simulink model "LOG_DATI_GPS_BMP_prova"  (R2020b)
settings: Solver=ode4  StartTime=0.0  StopTime=Inf  FixedStep=0.02  RelTol=1e-3  EnableMultiTasking=on
PostLoadFcn:
  | , if any(exist('dsrtsu_mdlpostloadfcn', 'file') == [2, 3, 6]), try dsrtsu_mdlpostloadfcn('Execute', bdroot); catch fprintf('Error in PostLoadFcn (dsrtsu_mdlpostloadfcn) for model "%s":\n %s\n', bdroot, lasterr); end, end,
InitFcn:
  | , if any(exist('rtifpga_mdlclblib', 'file') ~= 0), rtifpga_mdlclblib('Init', bdroot); end,
values from neighbouring files (symbols this model uses):
  t_AP = 0.02    [AVVIO_AENEA_DATA.m]    (also in workspace_SFT.mat)
libraries: arduinolib x21, simulink_extras x6, svdutilitieslib x4, simulink x2
(part 2 of 3)

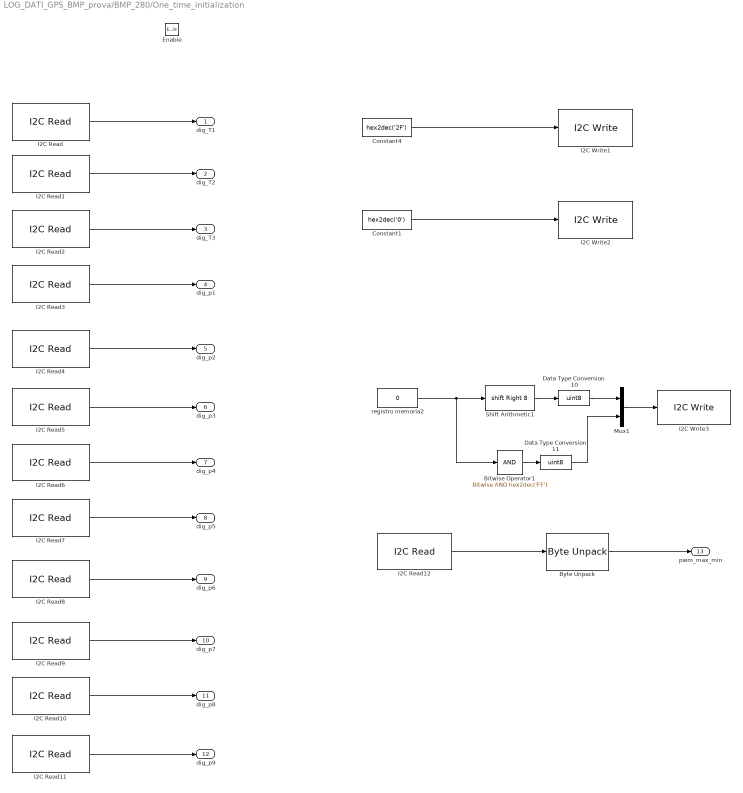
== system LOG_DATI_GPS_BMP_prova/BMP_280/One_time_initialization ==
  Enable : EnablePort
  Bitwise Operator1 : simulink/Logic and Bit Operations/Bitwise Operator  logicop=AND  UseBitMask=on  BitMask=hex2dec('FF')  BitMaskRealWorld=Stored Integer
  Byte Unpack : svdutilitieslib/Byte Unpack  dimensions={[8]}  datatypes={'uint16'}  byteAlign=1  blockPlatform=arduinoert
      settings: SourceProductBaseCode=ARDUINO
  Constant1 : Constant  Value=hex2dec('0')  OutDataTypeStr=uint8  SampleTime=-1
  Constant4 : Constant  Value=hex2dec('2F')  OutDataTypeStr=uint8  SampleTime=-1
  Data Type Conversion10 : DataTypeConversion  OutDataTypeStr=uint8
  Data Type Conversion11 : DataTypeConversion  OutDataTypeStr=uint8
  I2C Read : arduinolib/I2C Read  Priority=1  I2CModule=0  Mode=Master  SlaveAddress=hex2dec( '76' )  SlaveByteOrder=LittleEndian  Direction=Receiver  RegisterAddressMode=on  RegisterAddress=hex2dec( '88' )  SlaveDataType=uint16  DataLength=1  NoAck=off  RepeatedStart=off  OutputStatus=off  blockPlatform=arduino  SampleTime=t_AP
      settings: AttributesFormatString=Priority=%<Priority>  SourceProductBaseCode=ARDUINO
  I2C Read1 : arduinolib/I2C Read  Priority=2  I2CModule=0  Mode=Master  SlaveAddress=hex2dec( '76' )  SlaveByteOrder=LittleEndian  Direction=Receiver  RegisterAddressMode=on  RegisterAddress=hex2dec( '8A' )  SlaveDataType=int16  DataLength=1  NoAck=off  RepeatedStart=off  OutputStatus=off  blockPlatform=arduino  SampleTime=t_AP
      settings: AttributesFormatString=Priority=%<Priority>  SourceProductBaseCode=ARDUINO
  I2C Read10 : arduinolib/I2C Read  Priority=11  I2CModule=0  Mode=Master  SlaveAddress=hex2dec( '76' )  SlaveByteOrder=LittleEndian  Direction=Receiver  RegisterAddressMode=on  RegisterAddress=hex2dec( '9C' )  SlaveDataType=int16  DataLength=1  NoAck=off  RepeatedStart=off  OutputStatus=off  blockPlatform=arduino  SampleTime=t_AP
      settings: AttributesFormatString=Priority=%<Priority>  SourceProductBaseCode=ARDUINO
  I2C Read11 : arduinolib/I2C Read  Priority=12  I2CModule=0  Mode=Master  SlaveAddress=hex2dec( '76' )  SlaveByteOrder=LittleEndian  Direction=Receiver  RegisterAddressMode=on  RegisterAddress=hex2dec( '9E' )  SlaveDataType=int16  DataLength=1  NoAck=off  RepeatedStart=off  OutputStatus=off  blockPlatform=arduino  SampleTime=t_AP
      settings: AttributesFormatString=Priority=%<Priority>  SourceProductBaseCode=ARDUINO
  I2C Read12 : arduinolib/I2C Read  Priority=16  I2CModule=0  Mode=Master  SlaveAddress=hex2dec( '50' )  SlaveByteOrder=BigEndian  Direction=Receiver  RegisterAddressMode=off  RegisterAddress=0  SlaveDataType=uint8  DataLength=16  NoAck=off  RepeatedStart=off  OutputStatus=off  blockPlatform=ARDUINO  SampleTime=0.02
      settings: AttributesFormatString=Priority=%<Priority>  SourceProductBaseCode=ARDUINO
  I2C Read2 : arduinolib/I2C Read  Priority=3  I2CModule=0  Mode=Master  SlaveAddress=hex2dec( '76' )  SlaveByteOrder=LittleEndian  Direction=Receiver  RegisterAddressMode=on  RegisterAddress=hex2dec( '8C' )  SlaveDataType=int16  DataLength=1  NoAck=off  RepeatedStart=off  OutputStatus=off  blockPlatform=arduino  SampleTime=t_AP
      settings: AttributesFormatString=Priority=%<Priority>  SourceProductBaseCode=ARDUINO
  I2C Read3 : arduinolib/I2C Read  Priority=4  I2CModule=0  Mode=Master  SlaveAddress=hex2dec( '76' )  SlaveByteOrder=LittleEndian  Direction=Receiver  RegisterAddressMode=on  RegisterAddress=hex2dec( '8E' )  SlaveDataType=uint16  DataLength=1  NoAck=off  RepeatedStart=off  OutputStatus=off  blockPlatform=arduino  SampleTime=t_AP
      settings: AttributesFormatString=Priority=%<Priority>  SourceProductBaseCode=ARDUINO
  I2C Read4 : arduinolib/I2C Read  Priority=5  I2CModule=0  Mode=Master  SlaveAddress=hex2dec( '76' )  SlaveByteOrder=LittleEndian  Direction=Receiver  RegisterAddressMode=on  RegisterAddress=hex2dec( '90' )  SlaveDataType=int16  DataLength=1  NoAck=off  RepeatedStart=off  OutputStatus=off  blockPlatform=arduino  SampleTime=t_AP
      settings: AttributesFormatString=Priority=%<Priority>  SourceProductBaseCode=ARDUINO
  I2C Read5 : arduinolib/I2C Read  Priority=6  I2CModule=0  Mode=Master  SlaveAddress=hex2dec( '76' )  SlaveByteOrder=LittleEndian  Direction=Receiver  RegisterAddressMode=on  RegisterAddress=hex2dec( '92' )  SlaveDataType=int16  DataLength=1  NoAck=off  RepeatedStart=off  OutputStatus=off  blockPlatform=arduino  SampleTime=t_AP
      settings: AttributesFormatString=Priority=%<Priority>  SourceProductBaseCode=ARDUINO
  I2C Read6 : arduinolib/I2C Read  Priority=7  I2CModule=0  Mode=Master  SlaveAddress=hex2dec( '76' )  SlaveByteOrder=LittleEndian  Direction=Receiver  RegisterAddressMode=on  RegisterAddress=hex2dec( '94' )  SlaveDataType=int16  DataLength=1  NoAck=off  RepeatedStart=off  OutputStatus=off  blockPlatform=arduino  SampleTime=t_AP
      settings: AttributesFormatString=Priority=%<Priority>  SourceProductBaseCode=ARDUINO
  I2C Read7 : arduinolib/I2C Read  Priority=8  I2CModule=0  Mode=Master  SlaveAddress=hex2dec( '76' )  SlaveByteOrder=LittleEndian  Direction=Receiver  RegisterAddressMode=on  RegisterAddress=hex2dec( '96' )  SlaveDataType=int16  DataLength=1  NoAck=off  RepeatedStart=off  OutputStatus=off  blockPlatform=arduino  SampleTime=t_AP
      settings: AttributesFormatString=Priority=%<Priority>  SourceProductBaseCode=ARDUINO
  I2C Read8 : arduinolib/I2C Read  Priority=9  I2CModule=0  Mode=Master  SlaveAddress=hex2dec( '76' )  SlaveByteOrder=LittleEndian  Direction=Receiver  RegisterAddressMode=on  RegisterAddress=hex2dec( '98' )  SlaveDataType=int16  DataLength=1  NoAck=off  RepeatedStart=off  OutputStatus=off  blockPlatform=arduino  SampleTime=t_AP
      settings: AttributesFormatString=Priority=%<Priority>  SourceProductBaseCode=ARDUINO
  I2C Read9 : arduinolib/I2C Read  Priority=10  I2CModule=0  Mode=Master  SlaveAddress=hex2dec( '76' )  SlaveByteOrder=LittleEndian  Direction=Receiver  RegisterAddressMode=on  RegisterAddress=hex2dec( '9A' )  SlaveDataType=int16  DataLength=1  NoAck=off  RepeatedStart=off  OutputStatus=off  blockPlatform=arduino  SampleTime=t_AP
      settings: AttributesFormatString=Priority=%<Priority>  SourceProductBaseCode=ARDUINO
  I2C Write1 : arduinolib/I2C Write  Priority=13  I2CModule=0  Mode=Master  SlaveAddress=hex2dec( '76' )  SlaveByteOrder=LittleEndian  Direction=Transmitter  RegisterAddressMode=on  RegisterAddress=hex2dec( 'F4' )  SlaveDataType=uint8  DataLength=1  NoAck=off  RepeatedStart=off  OutputStatus=off  blockPlatform=arduino
      settings: AttributesFormatString=Priority=%<Priority>  SourceProductBaseCode=ARDUINO
  I2C Write2 : arduinolib/I2C Write  Priority=14  I2CModule=0  Mode=Master  SlaveAddress=hex2dec( '76' )  SlaveByteOrder=LittleEndian  Direction=Transmitter  RegisterAddressMode=on  RegisterAddress=hex2dec( 'F5' )  SlaveDataType=uint8  DataLength=1  NoAck=off  RepeatedStart=off  OutputStatus=off  blockPlatform=arduino
      settings: AttributesFormatString=Priority=%<Priority>  SourceProductBaseCode=ARDUINO
  I2C Write3 : arduinolib/I2C Write  Priority=15  I2CModule=0  Mode=Master  SlaveAddress=hex2dec( '50' )  SlaveByteOrder=BigEndian  Direction=Transmitter  RegisterAddressMode=off  RegisterAddress=hex2dec( '0' )  SlaveDataType=uint8  DataLength=1  NoAck=off  RepeatedStart=off  OutputStatus=off  blockPlatform=ARDUINO
      settings: AttributesFormatString=Priority=%<Priority>  SourceProductBaseCode=ARDUINO
  Mux1 : Mux  Inputs=2
  Shift Arithmetic1 : ArithShift  BitShiftNumber=8  BitShiftDirection=Right
  "registro memoria2 " : Constant  Value=0  OutDataTypeStr=uint16  SampleTime=t_AP
  dig_T1 : Outport  VectorParamsAs1DForOutWhenUnconnected=off
  dig_T2 : Outport  Port=2  VectorParamsAs1DForOutWhenUnconnected=off
  dig_T3 : Outport  Port=3  VectorParamsAs1DForOutWhenUnconnected=off
  dig_p1 : Outport  Port=4  VectorParamsAs1DForOutWhenUnconnected=off
  dig_p2 : Outport  Port=5  VectorParamsAs1DForOutWhenUnconnected=off
  dig_p3 : Outport  Port=6  VectorParamsAs1DForOutWhenUnconnected=off
  dig_p4 : Outport  Port=7  VectorParamsAs1DForOutWhenUnconnected=off
  dig_p5 : Outport  Port=8  VectorParamsAs1DForOutWhenUnconnected=off
  dig_p6 : Outport  Port=9  VectorParamsAs1DForOutWhenUnconnected=off
  dig_p7 : Outport  Port=10  VectorParamsAs1DForOutWhenUnconnected=off
  dig_p8 : Outport  Port=11  VectorParamsAs1DForOutWhenUnconnected=off
  dig_p9 : Outport  Port=12  VectorParamsAs1DForOutWhenUnconnected=off
  pwm_max_min : Outport  Port=13  VectorParamsAs1DForOutWhenUnconnected=off
  wires:
  Byte Unpack/1 -> pwm_max_min/1
  Data Type Conversion11/1 -> Mux1/2
  "registro memoria2 "/1 -> Bitwise Operator1/1, Shift Arithmetic1/1
  Bitwise Operator1/1 -> Data Type Conversion11/1
  Mux1/1 -> I2C Write3/1
  Shift Arithmetic1/1 -> Data Type Conversion10/1
  Data Type Conversion10/1 -> Mux1/1
  I2C Read12/1 -> Byte Unpack/1
  Constant1/1 -> I2C Write2/1
  Constant4/1 -> I2C Write1/1
  I2C Read1/1 -> dig_T2/1
  I2C Read3/1 -> dig_p1/1
  I2C Read11/1 -> dig_p9/1
  I2C Read9/1 -> dig_p7/1
  I2C Read2/1 -> dig_T3/1
  I2C Read6/1 -> dig_p4/1
  I2C Read5/1 -> dig_p3/1
  I2C Read/1 -> dig_T1/1
  I2C Read4/1 -> dig_p2/1
  I2C Read10/1 -> dig_p8/1
  I2C Read7/1 -> dig_p5/1
  I2C Read8/1 -> dig_p6/1

== system LOG_DATI_GPS_BMP_prova/BMP_280/Subsystem ==
  T : Inport
  Cal_alt : Inport  Port=2
  T_01 : Inport  Port=3
  Constant : Constant  Value=15
  NotEqual : RelationalOperator  Operator=~=  OutDataTypeStr=boolean  RndMeth=Simplest
  Subsystem1 : Subsystem
  Switch : Switch  Criteria=u2 > Threshold
  Switch1 : Switch  Criteria=u2 > Threshold
  T_02 : Outport  VectorParamsAs1DForOutWhenUnconnected=off
  Cal_alt2 : Outport  Port=2  VectorParamsAs1DForOutWhenUnconnected=off
  wires:
  T_01/1 -> NotEqual/2, Switch1/1, Switch/3
  Switch1/1 -> T_02/1
  Switch/1 -> Switch1/3
  Constant/1 -> NotEqual/1
  Subsystem1/1(T_0) -> Switch/1, Switch/2
  NotEqual/1 -> Switch1/2
  Cal_alt/1 -> Cal_alt2/1, Subsystem1/Enable
  T/1 -> Subsystem1/1(T)

== system LOG_DATI_GPS_BMP_prova/Subsystem2/Subsystem ==
  In1 : Inport
  Enable : EnablePort
  Complex to Real-Imag : ComplexToRealImag  Output=Real
  MATLAB Function : MATLAB Function  TreatAsAtomicUnit=on
  Memory : Memory  InheritSampleTime=on
  Mux : Mux  Inputs=9
  Outport : Outport  VectorParamsAs1DForOutWhenUnconnected=off
  mario : Outport  Port=2  VectorParamsAs1DForOutWhenUnconnected=off
  wires:
  MATLAB Function/2(Long) -> Mux/2  "Long"
  Memory/1 -> MATLAB Function/2(out_prec)
  MATLAB Function/8(h_mean_sea) -> Mux/8  "h_mean_sea"
  MATLAB Function/3(V) -> Mux/3  "hor_speed"
  MATLAB Function/1(Lat) -> Mux/1  "Lat"
  Mux/1 -> Complex to Real-Imag/1
  MATLAB Function/9(h_WGS84) -> Mux/9  "h_WGS85"
  MATLAB Function/5(heading) -> Mux/5  "heading"
  MATLAB Function/6(fix_mode) -> Mux/6  "fix_GPS"
  MATLAB Function/4(Magnetic_declination) -> Mux/4
  MATLAB Function/7(n_sat) -> Mux/7
  Complex to Real-Imag/1 -> Memory/1, Outport/1
  In1/1 -> MATLAB Function/1(messaggio)
  MATLAB Function/10(indice_dimario) -> mario/1

== system LOG_DATI_GPS_BMP_prova/AIR TX/Enable /Chart/sendbyte ==
  note: sostituito con lo stesso blocco della V. R2015a il 29/1/2016
  bt : Inport  OutDataTypeStr=uint8
  n : Inport  Port=2
  f : TriggerPort  TriggerType=function-call  VariantControl=(inherit)
      settings: CopyFcn=Stateflow.SLINSF.SimulinkMan.removeBlockPreDeleteFcn  PreDeleteFcn=Stateflow.SLINSF.SimulinkMan.unsafePredeleteFcn
  Selector : Selector  InputPortWidth=264  IndexOptions=Index vector (port)  Indices=[1 3]  OutputSizes=1
  Serial Transmit : arduinolib/Serial Transmit  portNumber=2  sendmode=write  sendformat=Decimal  floatprecision=2  blockPlatform=arduino
  wires:
  Selector/1 -> Serial Transmit/1
  n/1 -> Selector/2
  bt/1 -> Selector/1

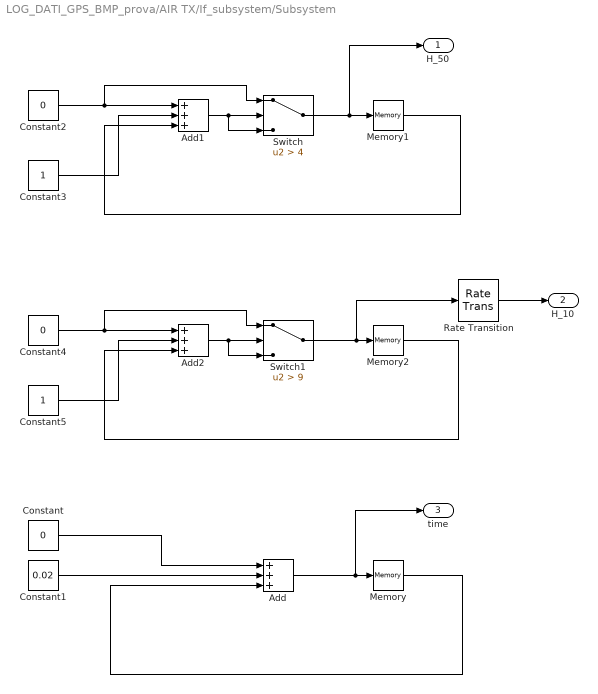
== system LOG_DATI_GPS_BMP_prova/AIR TX/If_subsystem/Subsystem ==
  Add : Sum  Inputs=+++
  Add1 : Sum  Inputs=+++
  Add2 : Sum  Inputs=+++
  Constant : Constant  Value=0  SampleTime=0.02
  Constant1 : Constant  Value=0.02  SampleTime=0.02
  Constant2 : Constant  Value=0  SampleTime=0.02
  Constant3 : Constant  SampleTime=0.02
  Constant4 : Constant  Value=0  SampleTime=0.02*5
  Constant5 : Constant  SampleTime=0.02*5
  Memory : Memory  InitialCondition=-0.02  InheritSampleTime=on
  Memory1 : Memory  InitialCondition=-1  InheritSampleTime=on
  Memory2 : Memory  InitialCondition=-1  InheritSampleTime=on
  Rate Transition : RateTransition  Deterministic=off  OutPortSampleTime=0.02
  Switch : Switch  Criteria=u2 > Threshold  Threshold=4
  Switch1 : Switch  Criteria=u2 > Threshold  Threshold=9
  H_50 : Outport  VectorParamsAs1DForOutWhenUnconnected=off
  H_10 : Outport  Port=2  VectorParamsAs1DForOutWhenUnconnected=off
  time : Outport  Port=3  VectorParamsAs1DForOutWhenUnconnected=off
  wires:
  Memory1/1 -> Add1/3
  Add2/1 -> Switch1/2, Switch1/3
  Constant4/1 -> Add2/1, Switch1/1
  Constant5/1 -> Add2/2
  Memory2/1 -> Add2/3
  Memory/1 -> Add/3
  Add/1 -> time/1, Memory/1
  Constant/1 -> Add/1
  Constant1/1 -> Add/2
  Constant2/1 -> Add1/1, Switch/1
  Switch/1 -> H_50/1, Memory1/1
  Constant3/1 -> Add1/2
  Add1/1 -> Switch/2, Switch/3
  Switch1/1 -> Rate Transition/1, Memory2/1
  Rate Transition/1 -> H_10/1

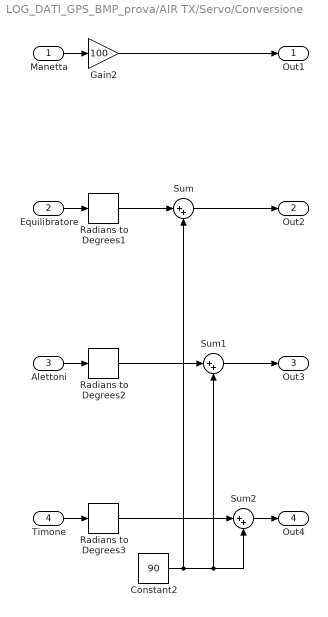
== system LOG_DATI_GPS_BMP_prova/AIR TX/Servo/Conversione ==
  Manetta : Inport
  Equilibratore : Inport  Port=2
  Alettoni : Inport  Port=3
  Timone : Inport  Port=4
  Constant2 : Constant  Value=90
  Gain2 : Gain  Gain=100
  Radians to Degrees1 : simulink_extras/Transformations/Radians to Degrees
  Radians to Degrees2 : simulink_extras/Transformations/Radians to Degrees
  Radians to Degrees3 : simulink_extras/Transformations/Radians to Degrees
  Sum : Sum  Inputs=|++
  Sum1 : Sum  Inputs=|++
  Sum2 : Sum  Inputs=|++
  Out1 : Outport  VectorParamsAs1DForOutWhenUnconnected=off
  Out2 : Outport  Port=2  VectorParamsAs1DForOutWhenUnconnected=off
  Out3 : Outport  Port=3  VectorParamsAs1DForOutWhenUnconnected=off
  Out4 : Outport  Port=4  VectorParamsAs1DForOutWhenUnconnected=off
  wires:
  Sum2/1 -> Out4/1
  Timone/1 -> Radians to Degrees3/1
  Sum1/1 -> Out3/1
  Alettoni/1 -> Radians to Degrees2/1
  Sum/1 -> Out2/1
  Equilibratore/1 -> Radians to Degrees1/1
  Gain2/1 -> Out1/1
  Manetta/1 -> Gain2/1
  Constant2/1 -> Sum2/2, Sum1/2, Sum/2
  Radians to Degrees3/1 -> Sum2/1
  Radians to Degrees2/1 -> Sum1/1
  Radians to Degrees1/1 -> Sum/1

== system LOG_DATI_GPS_BMP_prova/BMP_280/Subsystem/Subsystem1 ==
  T : Inport
  Enable : EnablePort
  T_0 : Outport  VectorParamsAs1DForOutWhenUnconnected=off
  wires:
  T/1 -> T_0/1

== matlab function LOG_DATI_GPS_BMP_prova/BMP_280/MATLAB Function ==
  data: rate_l_up output; Cal_alt input; P input; P_int input; P_refer output double; P_cal input; rate_l_dw output
function [rate_l_up, P_refer, rate_l_dw]  = fcn( Cal_alt, P,P_int,P_cal)
%#codegen

persistent P_ref rl_up rl_dw

if isempty(P_ref)
    
    P_ref = 101325;
    
end

if isempty(rl_up)
    
    rl_up = 300;
    
end

if isempty(rl_dw)
    
    rl_dw = -300;
    
end

if Cal_alt == 1
    
    P_ref = P;
 
end

if P_int == 1
   
   P_ref = P_cal; 
   rl_up = 20;
   rl_dw = -20;
    
end
    


P_refer = P_ref;

rate_l_up = rl_up;
rate_l_dw = rl_dw;

== matlab function LOG_DATI_GPS_BMP_prova/Subsystem2/Create_message ==
  data: status output; byte_pack input; messaggio output
function [status,messaggio]  = LETTURA_NMEA(byte_pack)

persistent message counter start_found end_found

status = false;       %ho aggiunto questo
messaggio = uint8(zeros(1,80)) ;
pos_end = uint8(0) ;
M = uint8(length(byte_pack)) ;


if isempty(end_found) 
    end_found = false ;
end 
if isempty(start_found) 
     start_found = false ;
end 
if isempty (counter) 
    counter = uint8(0) ;
end 
if isempty(message)
     message = uint8(zeros(1,80)) ;
end



if start_found == 0 
    for i = uint8(1) : M  
        if byte_pack(i) == '$' 
            message(1:M - (i-1)) = byte_pack(i:end) ;
            counter = M - (i-1) ; 
            start_found = true ;
            break
        end
    end
    
    
elseif start_found == 1
    for i = uint8(1) : M  
        if byte_pack(i) == 13 
            end_found = true ;
            pos_end = i ;
            break
        end
    end
    
    if end_found == 1
        message(counter + 1 : counter + pos_end) = byte_pack(1:pos_end) ;
        status = true;       %ho aggiunto questo
        messaggio = message ;
        end_found = false ;
        counter = M - pos_end ;
        if pos_end == M 
            start_found = false ; 
            message = uint8(zeros(1,80)) ;
        else  
            start_found = true ;
            message(1:(M - pos_end)) = byte_pack(pos_end + 1 : end) ;
            message(M - pos_end +1 : 80) = uint8(zeros(1,80 - (M - pos_end) )) ;
        end
         

    else 
    message(counter + 1 : M + counter ) = byte_pack ;
    counter = M + counter  ;
   
    end
    
    
 
        
    
    
end

== matlab function LOG_DATI_GPS_BMP_prova/Subsystem2/Subsystem/MATLAB Function ==
  data: messaggio input; Lat output; Long output; V output; Magnetic_declination output; heading output; fix_mode output; n_sat output; h_mean_sea output; h_WGS84 output; out_prec input; indice_dimario output
function [Lat,Long,V,Magnetic_declination,heading,fix_mode,n_sat,h_mean_sea,h_WGS84,indice_dimario] = parser_NMEA(messaggio,out_prec)
    

messaggio = char(messaggio) ;

comma_gga = uint8(zeros(1,14));
comma_rmc = uint8(zeros(1,12));
star = uint8(0);
dollar = uint8(0);
find_dollar = uint8(0);
find_comma = uint8(0);
message_type = uint8(zeros(1,5));
indice_dimario = uint8(0);





for i=1:length(messaggio)
   if messaggio(i) == '$'
       find_dollar = find_dollar + uint8(1);
   end
   if messaggio(i) == ','
       find_comma = find_comma + uint8(1);
   end
end
    
if (find_dollar == 1 && (find_comma == 12 || find_comma == 14))               % controllo se il numero di $ e , sono corretti all'interno di messaggio
                                                                             % altrimenti il messaggio è corrotto ed in output mando i messaggi
                                                                             % precedenti
dollar= find(messaggio == '$',1);

mess_type = messaggio(dollar(1) + 1 : dollar(1) + 5);                              % è il nome del messaggio arrivato

% decodifica mesaggio RMC

if mess_type == 'GPRMC'
comma_rmc = find(messaggio == ',');                                              % restituisce le posizioni delle virgole all'interno del messaggio
star = find(messaggio == '*');                                               % restituisce la posizione dell'asterisco all'interno del messaggio
dollar = find(messaggio == '$');                                             % restituisce la posizione del dollaro all'interno del messaggio

Lat_1 = str2double(messaggio(comma_rmc(3) + 1 : comma_rmc(3) + 2));
Lat_2 = str2double(messaggio(comma_rmc(3) + 3 : comma_rmc(4) - 1))/60;
Lat = Lat_1 + Lat_2;
if messaggio(comma_rmc(4) + 1) == 'S'
Lat = -Lat; 
end

Long_1 = str2double(messaggio(comma_rmc(5) + 1 : comma_rmc(5) + 3));
Long_2 = str2double(messaggio(comma_rmc(5) + 4 : comma_rmc(6) - 1))/60;
Long = Long_1 + Long_2;
if messaggio(comma_rmc(6) + 1) == 'W'
Long = -Long; 
end

V = str2double(messaggio(comma_rmc(7) + 1 : comma_rmc(8) - 1)); 
    
heading = str2double(messaggio(comma_rmc(8) + 1 : comma_rmc(9) - 1));

Magnetic_declination = str2double(messaggio(comma_rmc(10) + 1 : comma_rmc(11) - 1));
if messaggio(comma_rmc(11) + 1) == 'W'
Magnetic_declination = -Magnetic_declination; 
end

% questi dati non sono presenti nel messaggio rmc, quindi prendo quelli
% precedenti

fix_mode = complex(out_prec(6),0);

n_sat = complex(out_prec(7),0) ;

h_mean_sea = complex(out_prec(8),0) ;

h_WGS84 = complex(out_prec(9),0) ;


%%%%%%%%%%%%%%%%%%%%%%%%%%%%%%%%%%%%%%%%%%%%%%%%%%%%%%%%%

% calcolo checksum

ck_ric = char(zeros(1,2)) ;
ck_ric(1) = messaggio(star(1) + uint8(1))  ;
ck_ric(2) = messaggio(star(1) + uint8(2)) ;

NMEA_rmc_string = uint8(messaggio(dollar(1)+1:star(1)-1)) ;

checksum = uint8(0) ;
for i = 1:length(NMEA_rmc_string) 
    checksum = bitxor(checksum,NMEA_rmc_string(i),'uint8') ;
end

if checksum ~= hex2dec(ck_ric) 
    Lat = out_prec(1) ;
    Long = out_prec(2) ;
    V = out_prec(3) ;
    Magnetic_declination = out_prec(4);
    heading = out_prec(5) ; 
    fix_mode = complex(out_prec(6),0);
    n_sat = complex(out_prec(7),0) ;
    h_mean_sea = complex(out_prec(8),0) ;
    h_WGS84 = complex(out_prec(9),0) ;
    indice_dimario = uint8(10);
end

%%%%%%%%%%%%%%%%%%%%%%%%%%%%%%%%%%%%%%%%%%%%%%%%%%%%%%%%%%%

% decodifica mesaggio GGA

elseif mess_type == 'GPGGA'
comma_gga = find(messaggio == ','); 
star = find(messaggio == '*');
dollar = find(messaggio == '$');


Lat_1 = str2double(messaggio(comma_gga(2) + 1 : comma_gga(2) + 2));
Lat_2 = str2double(messaggio(comma_gga(2) + 3 : comma_gga(3) - 1))/60;
Lat = Lat_1 + Lat_2;
if messaggio(comma_gga(3) + 1) == 'S'
Lat = -Lat; 
end


Long_1 = str2double(messaggio(comma_gga(4) + 1 : comma_gga(4) + 3));
Long_2 = str2double(messaggio(comma_gga(4) + 4 : comma_gga(5) - 1))/60;
Long = Long_1 + Long_2;
if messaggio(comma_gga(5) + 1) == 'W'
Long = -Long; 
end


fix_mode = str2double(messaggio(comma_gga(6) + 1)); 

n_sat = str2double(messaggio(comma_gga(7) + 1 : comma_gga(8) - 1));

h_mean_sea = str2double(messaggio(comma_gga(9) + 1 : comma_gga(10) - 1));

h_WGS84 = str2double(messaggio(comma_gga(11) + 1 : comma_gga(12) - 1));

% questi dati non sono presenti nel messaggio rmc, quindi prendo quelli
% precedenti

V = out_prec(3) ;

Magnetic_declination = out_prec(4);

heading = out_prec(5) ; 

%%%%%%%%%%%%%%%%%%%%%%%%%%%%%%%%%%%%%%%%%%%%%%%%%%%%%%%%%%%%%%%%%%%

% calcolo del checksum
ck_ric = char(zeros(1,2)) ;
ck_ric(1) = messaggio(star(1) + uint8(1))  ;
ck_ric(2) = messaggio(star(1) + uint8(2)) ;

NMEA_gga_string = uint8(messaggio(dollar(1)+1:star(1)-1)) ;

checksum = uint8(0) ;
for i = 1:length(NMEA_gga_string) 
    checksum = bitxor(checksum,NMEA_gga_string(i),'uint8') ;
end

if checksum ~= hex2dec(ck_ric) 
    Lat = out_prec(1) ;
    Long = out_prec(2) ;
    V = out_prec(3) ;
    Magnetic_declination = out_prec(4);
    heading = out_prec(5) ; 
fix_mode = complex(out_prec(6),0);

n_sat = complex(out_prec(7),0) ;

h_mean_sea = complex(out_prec(8),0) ;

h_WGS84 = complex(out_prec(9),0) ;
indice_dimario = uint8(20);
   
    
end

%%%%%%%%%%%%%%%%%%%%%%%%%%%%%%%%%%%%%%%%%%%%%%%%%%%%%%%%%%%%%%%%%%%%
        
else
    
    Lat = out_prec(1) ;
    Long = out_prec(2) ;
    V = out_prec(3) ;
    Magnetic_declination = out_prec(4);
    heading = out_prec(5) ; 
fix_mode = complex(out_prec(6),0);

n_sat = complex(out_prec(7),0) ;

h_mean_sea = complex(out_prec(8),0) ;

h_WGS84 = complex(out_prec(9),0) ; 
   
    
    
end


else
    
    Lat = out_prec(1) ;
    Long = out_prec(2) ;
    V = out_prec(3) ;
    Magnetic_declination = out_prec(4);
    heading = out_prec(5) ; 
    fix_mode = complex(out_prec(6),0);
    n_sat = complex(out_prec(7),0) ;
    h_mean_sea = complex(out_prec(8),0) ;
    h_WGS84 = complex(out_prec(9),0) ; 
end

end

== stateflow chart LOG_DATI_GPS_BMP_prova/AIR TX/Enable /Chart ==
  state sendbyte(bt,n) [function]
  state Inputblock
    entry: i=1;
    Inputblock -> (junction 28)
    (junction 32) -> (junction 28) [order 1] : [ i<Len]
        | {i++;}
    (junction 28) -> (junction 32) : {sendbyte(datain,i);}
    (junction 32) -> (junction 48) [order 2] : {i=1;}
  (default) -> Inputblock
  data: bt function_input uint8; n function_input; datain input uint8; Len input uint16 size=1; i local uint8 =0

== matlab function LOG_DATI_GPS_BMP_prova/AIR TX/Heartbeat/Alarm set ==
  data: Alarm input; H_mav output; Rx_mode input

%%

function H_mav = Allarm_set(Alarm, Rx_mode)
%#cambia lo stato se c'è un allarme attivo
% Allarm: possibili allarmi proveniente dall'autopilota
% Rx_mode: richiesta da parte della stazione di terra
% H_mav: setto i parametri Base_mode e System_status del Heartbeat


H_mav = uint8(Rx_mode); % setta la modalità con quella ricevuta da terra

% se un allarme si attiva ha la precedenza sulla richiesta della QGC

if Alarm(1) == 1 % ovvero l'aereo è entrato in safe e si pone su traettoria circolare di sicurezza
    
    H_mav(1) = uint8(220); % MAV_MODE_AUTO_ARMED
    H_mav(2) = uint8(5);   % MAV_STATE_CRITICAL
%     H_mav(3) = uint8(128); % MAV_MODE_FLAG_SAFETY_ARMED

end

% se l'allareme di intervento pilota è attivo ha precedenza sull'allarm
% sefe per cui bisogna riscrivere lo stato del pilota

if Alarm(2) == 1 % si è attivato l'allarme dell'intervento pilota 
    
    H_mav(1) = uint8(216); % MAV_MODE_GUIDED_ARMED
    H_mav(2) = uint8(4);   % MAV_STATE_ACTIVE
%     H_mav(3) = uint8(8);   % MAV_MODE_FLAG_GUIDED_ENABLED

end

== matlab function LOG_DATI_GPS_BMP_prova/AIR TX/If_subsystem/iflogic_function ==
  data: H50 input; iflogic output; H10 input
function iflogic = fcn(H50,H10)
%#codegen
% prende in ingeresso i counter che contano il tempo
% e dice quale messaggio bisogna inviare in base alle frequenze scelte in
% Heartbeat:            1Hz
% SCALED_IMU:           20Hz
%attitude:              20Hz
%GLOBAL_POSITION_INT:   1Hz
%SYS_STATUS:            3Hz
%VFR_HUD:               2Hz
%SERVO_OUTPUT_RAW       1Hz
%SCALED_PRESSURE        1Hz

if H50 == 1  || H50==3
    iflogic=uint8(26); % SCALED_IMU 20Hz
elseif H50==2 || H50==4
    iflogic=uint8(30); %attitude 20Hz
elseif  H50==0 && H10==2
    iflogic=uint8(33); %GLOBAL_POSITION_INT 1Hz
elseif  H50==0 && H10==6
    iflogic=uint8(34); %GLOBAL_POSITION_INT_RAW 1Hz
elseif  H50==0 && H10==0
    iflogic=uint8(0); %Heartbeat 1Hz
elseif H50==0 && (H10==1 || H10==5 || H10==9)
    iflogic=uint8(1); %SYS_STATUS 3Hz
elseif H50==0 && (H10==3 || H10==8)
    iflogic=uint8(74); %VFR_HUD 2Hz
elseif H50==0 && (H10==7)
    iflogic=uint8(36); %SERVO_OUTPUT_RAW 1Hz
elseif H50==0 && (H10==4)
    iflogic=uint8(29); %SCALED_PRESSURE 1Hz
else
    iflogic=uint8(255); %non esiste nessun messaggio con questo codice
    
end

== matlab function LOG_DATI_GPS_BMP_prova/AIR TX/Waypoints/MATLAB Function ==
  data: WP_info_in input; WP_param_in input; WP_info output; GC_info input; WP_param output
function [WP_info,WP_param] = fcn(WP_info_in,WP_param_in, GC_info)
%#codegen
WP_info=WP_info_in(1,:); %%per sicurezza
WP_param=WP_param_in(1,:); %%per sicurezza
[m,n]=size(WP_info_in);
if GC_info(1)==2
    if GC_info(2)>=0 && GC_info(2)<m %per poter inviare i MISSION_ITEM
        WP_info=WP_info_in(GC_info(2)+1,:);
        WP_param=WP_param_in(GC_info(2)+1,:);
    end
end
if GC_info(1)==3 && GC_info(2)>=0 && GC_info(2)<200 %per poter inviae i MISSION_REQUEST
    WP_info=WP_info_in(GC_info(2)+1,:);
end

== matlab function LOG_DATI_GPS_BMP_prova/BMP_280/MATLAB Function1 ==
  data: T_0 input; P_ref input; h_ output; P input
function h_  = fcn( T_0, P_ref,P)

%#codegen

g     = 9.81;    %accelerazione di gravità

R_gas = 287.05;  %costante dei gas perfetti

dTdh  = -0.0065; %gradiente termico verticale in atmosfera standard 

T_0        = T_0+273.15;


h_ = -1/(0.00012)*log(P/P_ref);

% h_ = ((R_gas/g)*log(P_ref/P)*T_0)/(1-(dTdh*0.5*(R_gas/g)*log(P_ref/P)));

== matlab function LOG_DATI_GPS_BMP_prova/AIR RX/MATLAB Function1 ==
  data: Base_mode input; GC_req input; value_c input; WP_info_in input; WP_param_in input; mem_out input; T_number input; T_ref input; Mav_state input; AP_int output; AP_rif output; H_mav output; SyS_data output; GC_info output; WP_db_out output; WP_db_param output; WP_AL output; Val_out_MAV output; T_0 output; AP_int_mem input; Base_mode_to_SF output; test output
function [AP_int, AP_rif, H_mav, SyS_data, GC_info, WP_db_out, WP_db_param,WP_AL, Val_out_MAV, T_0, Base_mode_to_SF, test] =...
    RXelaborazione(Base_mode, GC_req, value_c, WP_info_in, WP_param_in, mem_out, T_number, T_ref, Mav_state, AP_int_mem)
%#codegen
% PARTE PER LA GESTIONE DELLE RICHIESTE DALLA STAZIONE DI TERRA
% GC_req= richiesta della stazione di terra, vettore 2 componenti
%           GC_req(1)=1 :    inviare i parametri a fronte della ricezione del
%                           SET_Request
%                             se GC_req(2)=255 li invia tutti altrimenti
%                             solo 1
% value_c= valore da aggiornare;
% GC_info= necessario per S-function mavlink di trasmissione dipende dal
%               GC_req ricevuto
% WP_db_info= [WP_item255.count,WP_item255.seq,WP_item255.command,WP_item255.frame,
%               WP_item255.current,WP_info[5]=WP_item255.autocontinue]
% WP_db_param= parametri ultimo wp arrivato
% Val_out_MAV= valori aggiornati in uscita per il mavlink di trasmissione
% 
%  mem_out=[msg.sysid; msg.compid;msg.msgid;msg.len;msg.seq;flag]
%
% PARTE PER LA GESTIONE MANUALE AUTOMATICO
%Base_mode: richiesta da parte della stazione di terra di settare una
%           modalità di volo
%H_mav: setto i parametri Base_mode e System_status del Heartbeat di
%           trasmissione
%
%  VARIABILI NECESSARIE ALL'AUTOPILOTA
%AP_interruttori: interruttore di pilota automatico e manuale e modalità
%            [ manuale automatico HDG IAS ALT RC]
%
%AP_riferimenti: valori delle modalità di volo [HDG IAS ALT RC]

persistent riferimenti   % riferimenti delle modalità di volo
persistent WP_dbP WP_dbI WP_dbP_AL % lista dei parametri dei waypoint
persistent test1

nWPmax = uint16(6); % Numero massimo di WP da memorizzare %[MILONE]

% Inizializzazione

if isempty(riferimenti)
    
    riferimenti = single([0; 0; 0; 0; 0; 0; 0; 0; 20; 100; 2; 101325; 15; 0; 0; 0]) ; %valori di riferimento di ["I_HDG", "I_IAS", "I_ALT", "I_RC", "I_WP", "I_ATO", "I_AL" "V_HDG","V_IAS","V_ALT","V_RC","C_P0","C_T0","H_LAT","H_LONG","H_ALT"};]
    
end

if isempty(WP_dbP) || (GC_req(1) == 3 && GC_req(2) == 250)
    
        WP_dbP = single(zeros(nWPmax,7)); % nWPmax righe e 7 colonne
        WP_dbI = uint16(zeros(nWPmax,6)); % nWPmax righe e 6 colonne
        
        
end
if isempty(WP_dbP_AL) || (GC_req(1) == 3 && GC_req(2) == 250)                % introdotto da Sensolini: consente di inviare contemporaneamente wp di navigazione ed atterraggio
    
        WP_dbP_AL = single(zeros(nWPmax,7)); % nWPmax righe e 7 colonne
              
end

if isempty(test1)
    
    test1 = 0;
    
end


%% Parte di richieste da mavlik relativa al messaggio PARAM_SET

GC_info = [GC_req; mem_out(1)]; % GC_req (vettore di due) sarebbe GC_request nella S-Function ed è usato per la funzione di PARAM_SET; 
                                % mem_out(1) sarebbe nella S-Function mem_out[0]=msg.sysid; cioè chi interroga

if GC_info(1) == 1
    
    if GC_info(2) > 0 && GC_info(2) <= 7
        
        if abs(value_c) > 0 % attiva l'interruttore
            
            riferimenti(GC_info(2)) = single(1);
            
            %NB: se arrivano valori maggiori di 1 sempre 1 da in output perchè
            % gli interruttori possono essere solo di tipo 0/1
            % altrimenti l'autopilota si blocca
            
        elseif value_c == 0 % disattiva l'interruttore
            
            riferimenti(GC_info(2)) = single(0);
            
        end
        
    elseif GC_info(2) > 7 && GC_info(2) < 12
        
        riferimenti(GC_info(2)) = single(value_c);
        
    end
    
end

%% Parte relativa al messaggio COMMAND_LONG per la temperatura di riferimento dell'altimetro

if T_number == 13;
    
        riferimenti(T_number) = T_ref;
        
end

%%

Val_out_MAV = riferimenti; % output riferimenti

%% WP set

if GC_info(1) == 3 && GC_info(2) == 200 % arriva il numero dei waypoint
    
     if WP_info_in(1) > nWPmax  %%%ATTENZIONE!!  %[MILONE]
        WP_info_in(1) = nWPmax; % se nWP>nWPmax mi comporto come se avessi ricevuto solo i primi nWPmax
                                % non è ottimale, infatti QGC deve aspettare il time out, ma funziona
                                % va migliorata con una opportuna segnalazione
     end
     
     WP_dbI(:,1) = WP_info_in(1);
     
end

if GC_info(1) == 3 && GC_info(2) < 200 % è arrivato un waypoint
    
    if WP_param_in(2) == 0
    
    WP_dbP(WP_info_in(2)+1,:)   = single(WP_param_in); % 7Parametri. è arrivato il numero WP_info(2) +1 perchè in C si parte da 0
    WP_dbI(WP_info_in(2)+1,2:7) = WP_info_in(2:7);     % 6informazioni. è arrivato il numero WP_info(2)  +1 perchè in C si parte da 0
    
    else
     WP_dbP_AL(WP_param_in(1)+1,:) = single(WP_param_in);
     WP_dbI(WP_info_in(2)+1,2:7) = WP_info_in(2:7);
     
    end
    
end

WP_db_out   = WP_dbI;

WP_db_param = WP_dbP;
WP_AL = WP_dbP_AL;

%for i=1:WP_info_in(1)
%if WP_dbP(WP_info_in(2)+1,2) == 0
%    WP_db_param = WP_dbP;
%    WP_AL = single(zeros(nWPmax,7));
%else
%    WP_db_param = single(zeros(nWPmax,7));
%    WP_AL = WP_dbP;
%end
%end
%% parte di gestione modalità autopilota

H_mav   = uint8(zeros(2,1)); % inizializzo il vettore di output
AP_mode = uint8([0;0]);      % inizializzo il vettore che gli interrutori manuale e automatico

Base_mode_to_SF = uint8(0);

% setto i parametri necessari per l'hearbeat e per l'autopilota

if Base_mode == uint8(0) && Mav_state == uint8(0) % INIZIO: è la condizione che si verifica quando connetto Arduino a QGC, ovvero l'autopilota è in stato Standby
    
    H_mav(1) = uint8(0);         % MAV_MODE_PREFLIGHT
    H_mav(2) = uint8(3);         % MAV_STATE_STANDBY
%     H_mav(3) = uint8(64);        % MAV_MODE_FLAG_MANUAL_INPUT_ENABLED   %% il MAV_MODE_FLAG è commentato perché non lo utilizziamo dato che inviamo nel messaggio dell'heartbeat il MAV_MODE in corrispondenza del valore di base_mode (vedere la pagina web MAV'RIC)
    AP_mode  = uint8([1; 0]);    % attivo il manuale  spengo l'automatico
    Base_mode_to_SF = uint8(0);

elseif Base_mode == uint8(0) && Mav_state == uint8(3) % è arrivato MAV_MODE_PREFLIGHT e MAV_STATE_STANDBY (modalità Ready)
    
    H_mav(1) = uint8(0);         % MAV_MODE_PREFLIGHT
    H_mav(2) = uint8(3);         % MAV_STATE_STANDBY
%     H_mav(3) = uint8(64);        % MAV_MODE_FLAG_MANUAL_INPUT_ENABLED 
    AP_mode  = uint8([1; 0]);    % attivo il manuale  spengo l'automatico
    Base_mode_to_SF = uint8(0);
    test1 = 0;

elseif Base_mode == uint8(0) && Mav_state == uint8(2) % è arrivato MAV_MODE_PREFLIGHT e MAV_STATE_CALIBRATING
    
    H_mav(1) = uint8(0);         % MAV_MODE_PREFLIGHT
    H_mav(2) = uint8(2);         % MAV_STATE_CALIBRATING
%     H_mav(3) = uint8(64);        % MAV_MODE_FLAG_MANUAL_INPUT_ENABLED
    AP_mode  = uint8([1; 0]);    % attivo il manuale  spengo l'automatico
    Base_mode_to_SF = uint8(0);
    test1 = 0;
    
elseif Base_mode == uint8(0) && Mav_state == uint8(1) % è arrivato MAV_MODE_PREFLIGHT e MAV_STATE_BOOT
    
    H_mav(1) = uint8(0);         % MAV_MODE_PREFLIGHT
    H_mav(2) = uint8(1);         % MAV_STATE_BOOT
%     H_mav(3) = uint8(64);        % MAV_MODE_FLAG_MANUAL_INPUT_ENABLED
    AP_mode  = uint8([0; 1]);    % In questo caso si attiva l'interrutore di modalità automatica. 
                                 % Il motivo è dovuto al fatto che per fare la prova del safe è necessario che sia attivo 
                                 % il modo automatico altrimenti il safe non entra.
    Base_mode_to_SF = uint8(0);
    test1 = 1;
    
% elseif Base_mode==uint8(80)  %è arrivato MAV_MODE_STABILIZE_DISARMED, 1 manual in QGC
%     H_mav(1)=uint8(80);        %MAV_MODE_GUIDED_ARMED
%     H_mav(2)=uint8(4);          %MAV_STATE_ACTIVE
%     AP_mode=uint8([1; 0]);      %attivo il manuale  spengo l'automatico

elseif Base_mode == uint8(192) % è arrivato MAV_MODE_MANUAL_ARMED
    
    H_mav(1) = uint8(192);       % MAV_MODE_MANUAL_ARMED 
    H_mav(2) = uint8(4);         % MAV_STATE_ACTIVE
%     H_mav(3) = uint8(64);        % MAV_MODE_FLAG_MANUAL_INPUT_ENABLED
    AP_mode  = uint8([1; 0]);    % attivo il manuale  spengo l'automatico
    Base_mode_to_SF = uint8(192);
    
elseif Base_mode == uint8(208) % è arrivato MAV_MODE_STABILIZE_ARMED (sarebbe la modalità Stand By presente nello State Flow degli stati)
    
    H_mav(1) = uint8(208);       % MAV_MODE_STABILIZE_ARMED
    H_mav(2) = uint8(3);         % MAV_STATE_STANDBY
%     H_mav(3) = uint8(64);        % MAV_MODE_FLAG_MANUAL_INPUT_ENABLED
    AP_mode  = uint8([0; 0]);    % disattiva l'interruttore del manuale ma l'automatico non è ancora attivo
    Base_mode_to_SF = uint8(208);

elseif Base_mode == uint8(220) && Mav_state ~= uint8(5) % è arrivato MAV_MODE_AUTO_ARMED
    
    if (AP_int_mem(1) == uint8(0) && AP_int_mem(2) == uint8(0) && ((AP_int_mem(3) == uint8(1) || AP_int_mem(4) == uint8(1) ||...
        AP_int_mem(5) == uint8(1) || AP_int_mem(6) == uint8(1) || AP_int_mem(7) == uint8(1) || AP_int_mem(8) == uint8(1))))
    
        H_mav(1) = uint8(220);       % MAV_MODE_AUTO_ARMED
        H_mav(2) = uint8(4);         % MAV_STATE_ACTIVE
%         H_mav(3) = uint8(4);         % MAV_MODE_FLAG_AUTO_ENABLED
        AP_mode  = uint8([0; 1]);    % spengo il manuale attivo l'automatico
        Base_mode_to_SF = uint8(220);
        
    elseif (AP_int_mem(1) == uint8(0) && AP_int_mem(2) == uint8(1) && ((AP_int_mem(3) == uint8(1) || AP_int_mem(4) == uint8(1) ||...
            AP_int_mem(5) == uint8(1) || AP_int_mem(6) == uint8(1) || AP_int_mem(7) == uint8(1) || AP_int_mem(8) == uint8(1)))) 
        
        H_mav(1) = uint8(220);       % MAV_MODE_AUTO_ARMED
        H_mav(2) = uint8(4);         % MAV_STATE_ACTIVE
        AP_mode  = uint8([0; 1]);    % spengo il manuale attivo l'automatico
        Base_mode_to_SF = uint8(220);
        
    else 
        
        H_mav(1)  = uint8(208);       % MAV_MODE_STABILIZE_ARMED
        H_mav(2)  = uint8(3);         % MAV_STATE_STANDBY
        AP_mode   = uint8([0; 0]);    % attivo il manuale  spengo l'automatico
        Base_mode_to_SF = uint8(208);
    
    end

% elseif Base_mode == uint8(216)  % è arrivato MAV_MODE_GUIDED_ARMED
%     
%     H_mav(1) = uint8(8);         % MAV_MODE_FLAG_GUIDED_ENABLED
%     H_mav(2) = uint8(4);         % MAV_STATE_ACTIVE
%     AP_mode  = uint8([0; 1]);    % spengo il manuale attivo l'automatico
    
elseif Mav_state == uint8(5)  % si verifica nell'S-Function di ricezione quando il velivolo è andato in safe ovvero quando Alarm_Safe = 1
    
    H_mav(1) = uint8(220);      % MAV_MODE_AUTO_ARMED
    H_mav(2) = uint8(5);        % MAV_STATE_CRITICAL
%     H_mav(3) = uint8(128);      % MAV_MODE_FLAG_SAFETY_ARMED
    AP_mode  = uint8([0; 1]);   % spengo il manuale attivo l'automatico

% elseif Base_mode==uint8(66) % è arrivato MAV_MODE_TEST_DISARMED, lo usiamo per fare la calibrazione
%     H_mav(1)=uint8(64);        %MAV_MODE_FLAG_MANUAL_INPUT_ENABLED
%     H_mav(2)=uint8(2);         %MAV_STATE_CALIBRATING
%     AP_mode=uint8([1; 0]);     %attivo il manuale  spengo l'automatico
    
    %%%%%%%%%%%%%%%%%%%%%%%%%%%
    % elseif Base_mode==uint8(192) %%ARMED PREFLIGHT
    %     H_mav(1)=uint8(192);        %MAV_MODE_FLAG_MANUAL_INPUT_ENABLED
    %     H_mav(2)=uint8(3);          %	MAV_STATE_EMERGENCY
    %     AP_mode=uint8([0; 1]);     %spengo il manuale attivo l'automatico
    %     elseif Base_mode==uint8(64) %%DISARMED PREFLIGHT
    %     H_mav(1)=uint8(64);        %MAV_MODE_FLAG_MANUAL_INPUT_ENABLED
    %     H_mav(2)=uint8(3);          %	MAV_STATE_EMERGENCY
    %     AP_mode=uint8([0; 1]);     %spengo il manuale attivo l'automatico
    %     %%%%%%%%%%%%%%%%%%%%%%%%%%%%%%%%%%%%%%%

else
    
    H_mav(1) = uint8(192);       % MAV_MODE_MANUAL_ARMED 
    H_mav(2) = uint8(6);         % MAV_STATE_EMERGENCY
%     H_mav(3) = uint8(64);        % MAV_MODE_FLAG_MANUAL_INPUT_ENABLED
    AP_mode  = uint8([1; 0]);    % attivo il manuale  spengo l'automatico
    
end

%% parte delle informazioni sullo stato del sistema in ricezione

% calcolo dei messaggi persi provenienti dalla stazione di terra

drop_rate = 10*((100*mem_out(6))/mem_out(5));  % 10*percentuale !non moltipilicare direttamente per 10000 perchè è un uint16 e va in overflow
SyS_data  = [drop_rate mem_out(7) mem_out(3)];

%% parte per settare gli interrutori e i riferimenti

AP_int = [AP_mode; uint8(riferimenti(1:7))]; % interruttori
AP_rif = riferimenti(8:11);                  % riferimenti

T_0 = riferimenti(13); % valore della temperatura di riferimento T_0 dell'altimetro

test = test1;
